simulink model "moving_obj_tracking"  (R2019b)
settings: Solver=VariableStepAuto  StartTime=0.0  StopTime=75.0  RelTol=1e-3
undefined symbols (not defined in the file): objLabel, objX, sampleTime, targetLabel
libraries: mobileRoboticsLib x9, dspsrcs4 x1, robotalgslib x1
settings Model: Creator=kpera  LastModifiedBy=kpera

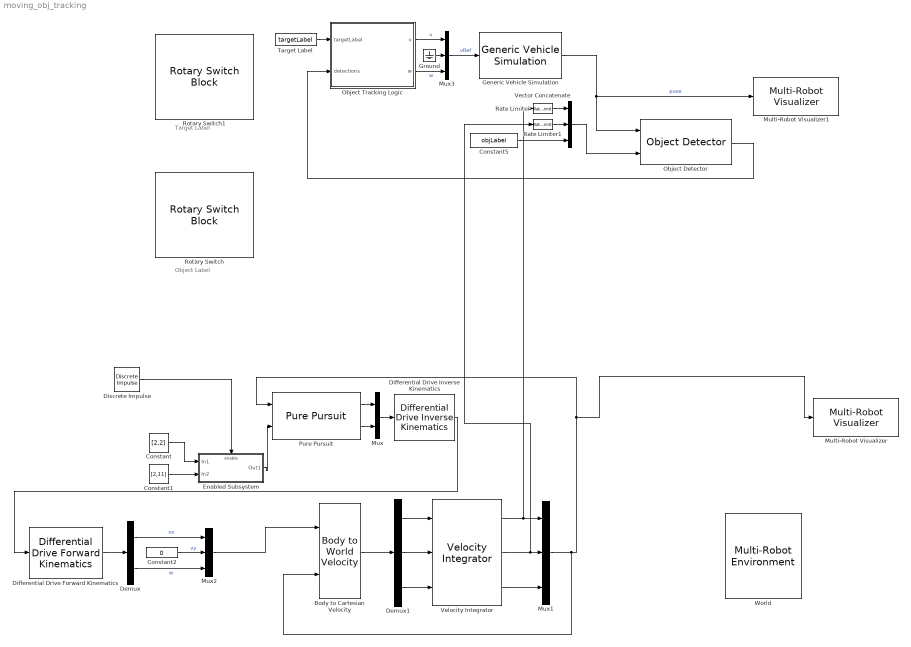
== system moving_obj_tracking ==
  note: Object Label
  note: Target Label
  Body to Cartesian Velocity : mobileRoboticsLib/Utilities/Body to World Velocity
      settings: SourceProductName=Mobile Robotics Simulation Toolbox
  Constant : Constant  Value=[2,2]  VectorParams1D=off
  Constant1 : Constant  Value=[2,11]  VectorParams1D=off
  Constant2 : Constant  Value=0
  Constant5 : Constant  Value=objLabel
  Demux : Demux  Outputs=2
  Demux1 : Demux  Outputs=3
  Differential Drive Inverse Kinematics : mobileRoboticsLib/Kinematic Models/Differential Drive/Differential Drive Inverse Kinematics  wheelRadius=0.1  wheelBase=0.5
      settings: SourceProductName=Mobile Robotics Simulation Toolbox
  Differential Drive Forward Kinematics : mobileRoboticsLib/Kinematic Models/Differential Drive/Differential Drive Forward Kinematics  wheelRadius=0.1  wheelBase=0.5
      settings: SourceProductName=Mobile Robotics Simulation Toolbox
  Discrete Impulse : dspsrcs4/Discrete  Impulse  Delay=0  SampleTime=1  FrameSample=1  OutputFrames=off  dataType=double  isSigned=on  wordLen=16  udDataType=sfix(16)  fracBitsMode=Best precision  numFracBits=15  OutDataTypeStr=double  LastOutDataTypeStr=double
  Enabled Subsystem : Subsystem  TreatAsAtomicUnit=on
  Generic Vehicle Simulation : mobileRoboticsLib/Utilities/Generic Vehicle Simulation  initX=2  initY=3  initAngle=0  Ts=sampleTime
      settings: SourceProductName=Mobile Robotics Simulation Library
  Ground : Ground
  Multi-Robot Visualizer : mobileRoboticsLib/Environments/Multi-Robot Visualizer  idx=1  radius=0  robotColor=[0 0 1]  showTraj=on  hasLidar=off  sensorOffset=[0,0]  scanAngles=[-pi/4, 0, pi/4]  hasObjDetector=off  objDetectorOffset=[0,0]  objDetectorAngle=0  objDetectorFOV=pi/3  objDetectorMaxRange=5
      settings: SourceProductName=Mobile Robotics Simulation Toolbox
  Multi-Robot Visualizer1 : mobileRoboticsLib/Environments/Multi-Robot Visualizer  idx=2  radius=0  robotColor=[0 0 1]  showTraj=on  hasLidar=off  sensorOffset=[0,0]  scanAngles=[-pi/4, 0, pi/4]  hasObjDetector=off  objDetectorOffset=[0,0]  objDetectorAngle=0  objDetectorFOV=pi/3  objDetectorMaxRange=5
      settings: SourceProductName=Mobile Robotics Simulation Toolbox
  Mux : Mux  Inputs=2
  Mux1 : Mux  Inputs=3
  Mux2 : Mux  Inputs=3
  Mux3 : Mux  Inputs=3
  Object Detector : mobileRoboticsLib/Environments/Object Detector  mapName=map  sensorOffset=objDetectorOffset  sensorAngle=objDetectorAngle  fieldOfView=objDetectorFOV  maxRange=objDetectorRange  maxDetections=objDetectorMaxHits  sampleTime=-1
      settings: SourceProductName=Ground Vehicles Library
  Object Tracking Logic : Stateflow chart  TreatAsAtomicUnit=on
  Pure Pursuit : robotalgslib/Pure Pursuit  DesiredLinearVelocity=0.15  MaxAngularVelocity=0.1  LookaheadDistance=0.35  TargetDirPort=off  SimulateUsing=Code generation
      settings: SourceProductName=Navigation Toolbox  SourceProductBaseCode=NV
  Rate Limiter : RateLimiter  SampleTimeMode=inherited  InitialCondition=objX
  Rate Limiter1 : RateLimiter  SampleTimeMode=inherited  InitialCondition=objX
  Rotary Switch : RotarySwitchBlock  LabelPosition=Hide
      settings: Values={{'RED', 'GREEN', 'BLUE'}, [1 2 3]}
  Rotary Switch1 : RotarySwitchBlock  LabelPosition=Hide
      settings: Values={{'RED', 'GREEN', 'BLUE'}, [1 2 3]}
  Target Label : Constant  Value=targetLabel
  Vector Concatenate : Concatenate  NumInputs=3  Mode=Multidimensional array  ConcatenateDimension=2
  Velocity Integrator : mobileRoboticsLib/Utilities/Generic Vehicle Simulation/Velocity Integrator  SystemSampleTime=-1  VariantControl=Variant1  LabelModeActiveChoice=mode==2  Latency=0  AutoFrameSizeCalculation=off
      link override Discrete/Discrete-Time Integrator: InitialCondition=2
      link override Discrete/Discrete-Time Integrator1: InitialCondition=2
      link override Discrete/Discrete-Time Integrator2: InitialCondition=90
      settings: SourceProductName=Mobile Robotics Simulation Toolbox
  World : mobileRoboticsLib/Environments/Multi-Robot Environment  numRobots=2  mapName=map  showWaypoints=off  showObjects=off  objectColors=[1 0 0;0 1 0;0 0 1]  objectMarkers='s'  showRobotIds=on  plotSensorLines=on
      settings: SourceProductName=Mobile Robotics Simulation Toolbox
  wires:
  Mux1/1 -> Multi-Robot Visualizer/1, Pure Pursuit/1, Body to Cartesian Velocity/2
  Pure Pursuit/2 -> Mux/2
  Mux/1 -> Differential Drive Inverse Kinematics/1
  Discrete Impulse/1 -> Enabled Subsystem/Enable
  Constant/1 -> Enabled Subsystem/1(In1)
  Pure Pursuit/1 -> Mux/1
  Enabled Subsystem/1(Out1) -> Pure Pursuit/2
  Constant1/1 -> Enabled Subsystem/2(In2)
  Demux1/1 -> Velocity Integrator/1
  Mux2/1 -> Body to Cartesian Velocity/1
  Demux1/3 -> Velocity Integrator/3
  Body to Cartesian Velocity/1 -> Demux1/1
  Demux1/2 -> Velocity Integrator/2
  Velocity Integrator/3 -> Mux1/3
  Demux/1 -> Mux2/1  "vx"
  Differential Drive Forward Kinematics/1 -> Demux/1
  Differential Drive Inverse Kinematics/1 -> Differential Drive Forward Kinematics/1
  Constant2/1 -> Mux2/2  "vy"
  Demux/2 -> Mux2/3  "w"
  Ground/1 -> Mux3/2
  Object Tracking Logic/2(w) -> Mux3/3  "w"
  Velocity Integrator/2 -> Rate Limiter1/1, Mux1/2
  Mux3/1 -> Generic Vehicle Simulation/1  "vRef"
  Rate Limiter1/1 -> Vector Concatenate/2
  Object Tracking Logic/1(v) -> Mux3/1  "v"
  Constant5/1 -> Vector Concatenate/3
  Velocity Integrator/1 -> Rate Limiter/1, Mux1/1
  Object Detector/1 -> Object Tracking Logic/2(detections)
  Target Label/1 -> Object Tracking Logic/1(targetLabel)
  Rate Limiter/1 -> Vector Concatenate/1
  Vector Concatenate/1 -> Object Detector/2
  Generic Vehicle Simulation/1 -> Multi-Robot Visualizer1/1, Object Detector/1  "pose"

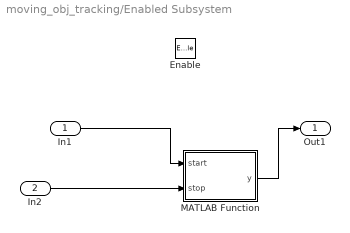
== system moving_obj_tracking/Enabled Subsystem ==
  In1 : Inport
  In2 : Inport  Port=2
  Enable : EnablePort  PropagateVarSize=During execution
  MATLAB Function : MATLAB Function  TreatAsAtomicUnit=on
  Out1 : Outport
  wires:
  In1/1 -> MATLAB Function/1(start)
  MATLAB Function/1(y) -> Out1/1
  In2/1 -> MATLAB Function/2(stop)

== matlab function moving_obj_tracking/Enabled Subsystem/MATLAB Function ==
  data: start input; y output size=[7,2] [..Inf]; stop input
function y = fcn(start, stop)
    path = [start,stop];
    flag = 1;
    while(flag == 1)
        s = load ('exampleMaps.mat');
        map = binaryOccupancyMap(s.simpleMap,2);
    %     R = 0.2;
    %     L = 0.1;
        map_inflate = copy(map);
        inflate(map_inflate,0.1)
        prm = mobileRobotPRM(map_inflate);
    %     prm.Map = map_inflate;
        prm.NumNodes = 50;
        prm.ConnectionDistance = 5;
        path = findpath(prm,start,stop);
        while isempty(path)
        % No feasible path found yet, increase the number of nodes
        prm.NumNodes = prm.NumNodes + 10;

        % Use the |update| function to re-create the PRM roadmap with the changed
        % attribute
        update(prm);

        % Search for a feasible path with the updated PRM
        path = findpath(prm, start, stop);
        end
        
        flag = 0;
    end
    y=path;
end

== stateflow chart moving_obj_tracking/Object Tracking Logic ==
  state TrackObject
    entry, during:
    [range,angle,valid] = findValidObject(targetLabel);
    if valid
    count = 0;
    else
    count = count + 1;
    end
    (default) -> (junction 20)
    TrackObject -> (junction 20) [order 1]
    (junction 20) -> (junction 24) [order 1] : % Set angular speed if
        | % angle outside deadband
        | [abs(angle) > pi/24]
    (junction 20) -> (junction 30) [order 2] : {w = 0;}
    (junction 24) -> (junction 49) : % Proportional
        | % control
        | {w = 1.5*angle;}
    (junction 49) -> (junction 30)
    (junction 30) -> (junction 54)
    (junction 54) -> (junction 56) [order 1] : % Go forward if object is far
        | [range > 1]
    (junction 54) -> (junction 60) [order 2] : {v = 0;}
    (junction 56) -> (junction 58) : {v = 0.5;}
    (junction 58) -> (junction 60)
  state SeekObject
    entry:
    v = 0;
    w = 1;
  (default) -> TrackObject : {
      | count = 0;
      | range = 0;
      | angle = 0;
      | }
  TrackObject -> SeekObject [order 1] : [count > 20]
  SeekObject -> TrackObject : [~isempty(detections)]
  data: dist function_output; ang function_output; flag function_output; label function_input; targetLabel input; detections input size=[objDetectorMaxHits,3]; v output; w output; angle local; range local; count local; valid local
  function [dist,ang,flag] = findValidObject(label):
    | function [dist,ang,flag] = findValidObject(label)
    | % Finds the distance (dist) and angle (ang) of the nearest valid
    | % object detected. If an object is found, the (flag) output is true.
    | 
    | % Initialize
    | flag = false;
    | dist = 0;
    | ang = 0;
    | 
    | if ~isempty(detections)
    |     % Loop through all detections
    |     for idx = 1:size(detections,1)
    |         % If a detection matching the target label is found, 
    |         % return it and set the valid flag to true.
    |         if detections(idx,3) == label
    |             dist = detections(idx,1);
    |             ang  = detections(idx,2);
    |             flag = true;
    |             return; 
    |         end
    |     end
    | end
